simulink model "Control_base"  (R2020a)
settings: Solver=FixedStepAuto  StartTime=0.0  StopTime=20.0  FixedStep=0.01  RelTol=1e-3
undefined symbols (not defined in the file or in its folder): H_b
settings Model: Creator=João Lula  LastModifiedBy=João Lula

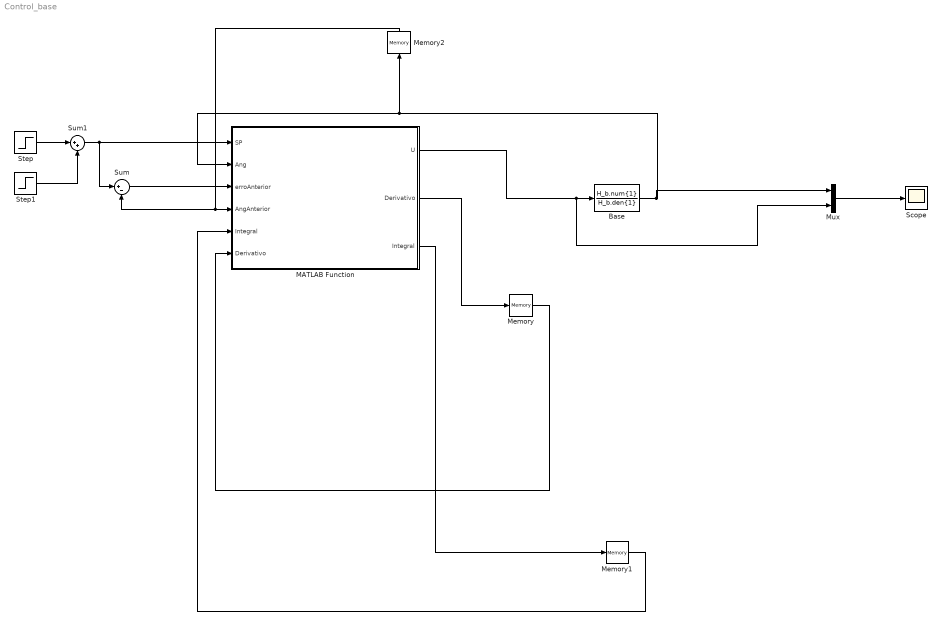
== system Control_base ==
  Base : TransferFcn  Numerator=H_b.num{1}  Denominator=H_b.den{1}
  MATLAB Function : MATLAB Function  TreatAsAtomicUnit=on
  Memory : Memory
  Memory1 : Memory
  Memory2 : Memory
  Mux : Mux  Inputs=2
  Scope : Scope
  Step : Step  Time=0  After=150  SampleTime=0
  Step1 : Step  Time=10  After=30  SampleTime=0
  Sum : Sum  Inputs=|+-
  Sum1 : Sum  Inputs=|++
  wires:
  MATLAB Function/1(U) -> Mux/2, Base/1
  MATLAB Function/2(Derivativo) -> Memory/1
  Memory/1 -> MATLAB Function/6("Derivativo ")
  MATLAB Function/3(Integral) -> Memory1/1
  Memory1/1 -> MATLAB Function/5("Integral ")
  Base/1 -> Mux/1, MATLAB Function/2(Ang), Memory2/1
  Memory2/1 -> Sum/2, MATLAB Function/4(AngAnterior)
  Sum/1 -> MATLAB Function/3(erroAnterior)
  Sum1/1 -> MATLAB Function/1(SP), Sum/1
  Step/1 -> Sum1/1
  Step1/1 -> Sum1/2
  Mux/1 -> Scope/1

== matlab function Control_base/MATLAB Function ==
  data: SP input; U output; Ang input; erroAnterior input; AngAnterior input; Integral input; Derivativo input; Derivativo output; Integral output
function [U, Derivativo, Integral] = PID(SP, Ang, erroAnterior, AngAnterior, Integral, Derivativo)


N = 100;

%% beta = 1
% K_c1 = 1.084;
% tau_i1 = 0.2353;
% taud_d1 = 0.0434;

%% beta = 2
% K_c1 = 0.7204;
% tau_i1 = 0.2300;
% taud_d1 = 0.0155;


%% beta = 5
K_c1 = 0.3687;
tau_i1 = 0.1900;
taud_d1 = 0.0011;

%% implementação do PID

Deltat = 0.01;


erro = SP - Ang;

Proporcional = K_c1 * erro;

Integral = Integral + (K_c1 * Deltat / tau_i1) * erroAnterior;

Derivativo = (taud_d1 / (taud_d1 + N * Deltat)) *Derivativo ...
               - ((K_c1 * taud_d1 * N) / (taud_d1 + N * Deltat)) * (Ang - AngAnterior);


U = Proporcional + Integral  + Derivativo;
end
